simulink model "PerturbacoesOrbitais"  (R2023b)
settings: Solver=FixedStepAuto  StartTime=0.0  StopTime=tf  FixedStep=step_modelo  RelTol=1e-3
values from neighbouring files (symbols this model uses):
  J2 = 1082.63E-6    (= 0.00108263)    [constantes.m]
  mi = 3.9860044189*10^14    (= 398600441890000)    [constantes.m]
  omega_E = 7.29211585530*10^-5    (= 7.2921158553e-05)    [constantes.m]
  Re = 6378.1363*10^3    (= 6378136.3)    [constantes.m]
undefined symbols (not defined in the file or in its folder): Cd0, Cd1, drag, J2_dist, L0, L1, m0, m1
settings Model: Creator=rodri  LastModifiedBy=rodri
settings DataIOCC: SaveOutput=off  SaveTime=off
settings ModelReferenceCC: EnableRefExpFcnMdlSchedulingChecks=on

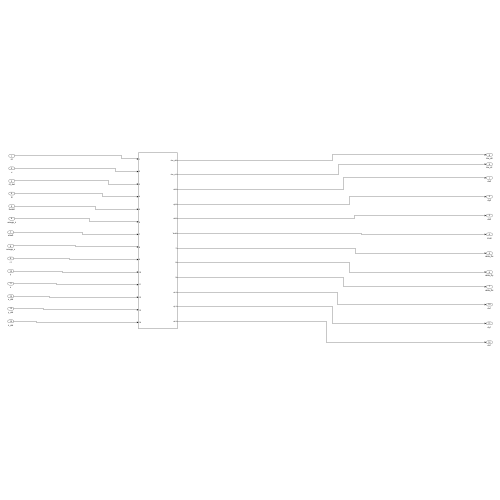
[thumbnail: Simulink's stored preview of the top-level diagram]
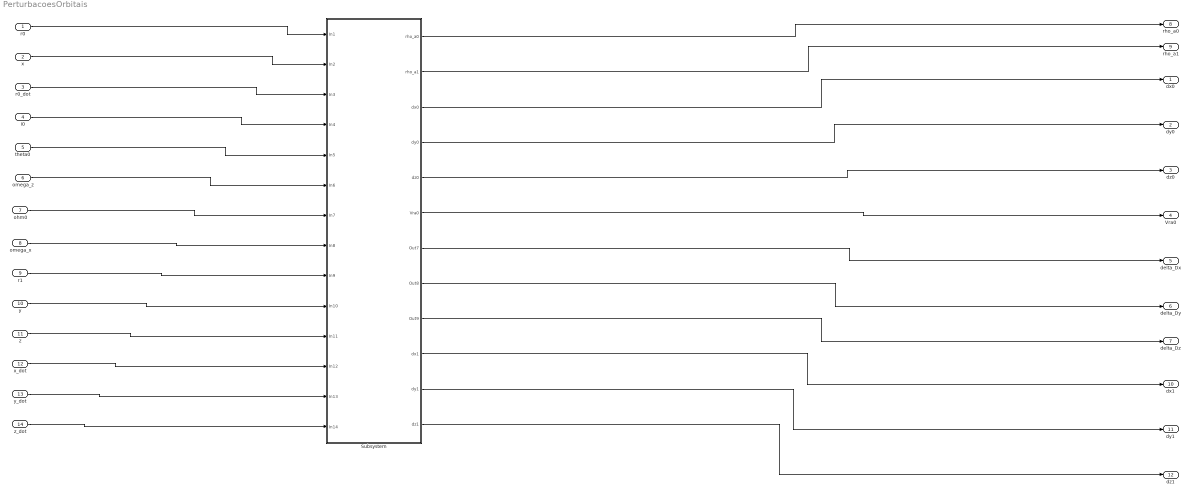
== system PerturbacoesOrbitais ==
  r0 : Inport  OutDataTypeStr=double  PortDimensions=1
  x : Inport  Port=2  OutDataTypeStr=double  PortDimensions=1
  r0_dot : Inport  Port=3  OutDataTypeStr=double  PortDimensions=1
  i0 : Inport  Port=4  OutDataTypeStr=double  PortDimensions=1
  theta0 : Inport  Port=5  OutDataTypeStr=double  PortDimensions=1
  omega_z : Inport  Port=6  OutDataTypeStr=double  PortDimensions=1
  ohm0 : Inport  Port=7  OutDataTypeStr=double  PortDimensions=1
  omega_x : Inport  Port=8  OutDataTypeStr=double  PortDimensions=1
  r1 : Inport  Port=9  OutDataTypeStr=double  PortDimensions=1
  y : Inport  Port=10  OutDataTypeStr=double  PortDimensions=1
  z : Inport  Port=11  OutDataTypeStr=double  PortDimensions=1
  x_dot : Inport  Port=12  OutDataTypeStr=double  PortDimensions=1
  y_dot : Inport  Port=13  OutDataTypeStr=double  PortDimensions=1
  z_dot : Inport  Port=14  OutDataTypeStr=double  PortDimensions=1
  Subsystem : Subsystem
  dx0 : Outport  OutDataTypeStr=double  PortDimensions=1
  dy0 : Outport  Port=2  OutDataTypeStr=double  PortDimensions=1
  dz0 : Outport  Port=3  OutDataTypeStr=double  PortDimensions=1
  Vra0 : Outport  Port=4  OutDataTypeStr=double  PortDimensions=1
  delta_Dx : Outport  Port=5  OutDataTypeStr=double  PortDimensions=1
  delta_Dy : Outport  Port=6  OutDataTypeStr=double  PortDimensions=1
  delta_Dz : Outport  Port=7  OutDataTypeStr=double  PortDimensions=1
  rho_a0 : Outport  Port=8  OutDataTypeStr=double  PortDimensions=1
  rho_a1 : Outport  Port=9  OutDataTypeStr=double  PortDimensions=1
  dx1 : Outport  Port=10  OutDataTypeStr=double  PortDimensions=1
  dy1 : Outport  Port=11  OutDataTypeStr=double  PortDimensions=1
  dz1 : Outport  Port=12  OutDataTypeStr=double  PortDimensions=1
  wires:
  r0/1 -> Subsystem/1(In1)
  x/1 -> Subsystem/2(In2)
  r0_dot/1 -> Subsystem/3(In3)
  i0/1 -> Subsystem/4(In4)
  theta0/1 -> Subsystem/5(In5)
  omega_z/1 -> Subsystem/6(In6)
  ohm0/1 -> Subsystem/7(In7)
  omega_x/1 -> Subsystem/8(In8)
  r1/1 -> Subsystem/9(In9)
  y/1 -> Subsystem/10(In10)
  z/1 -> Subsystem/11(In11)
  x_dot/1 -> Subsystem/12(In12)
  y_dot/1 -> Subsystem/13(In13)
  z_dot/1 -> Subsystem/14(In14)
  Subsystem/1(rho_a0) -> rho_a0/1
  Subsystem/2(rho_a1) -> rho_a1/1
  Subsystem/3(dx0) -> dx0/1
  Subsystem/4(dy0) -> dy0/1
  Subsystem/5(dz0) -> dz0/1
  Subsystem/6(Vra0) -> Vra0/1
  Subsystem/7(Out7) -> delta_Dx/1
  Subsystem/8(Out8) -> delta_Dy/1
  Subsystem/9(Out9) -> delta_Dz/1
  Subsystem/10(dx1) -> dx1/1
  Subsystem/11(dy1) -> dy1/1
  Subsystem/12(dz1) -> dz1/1

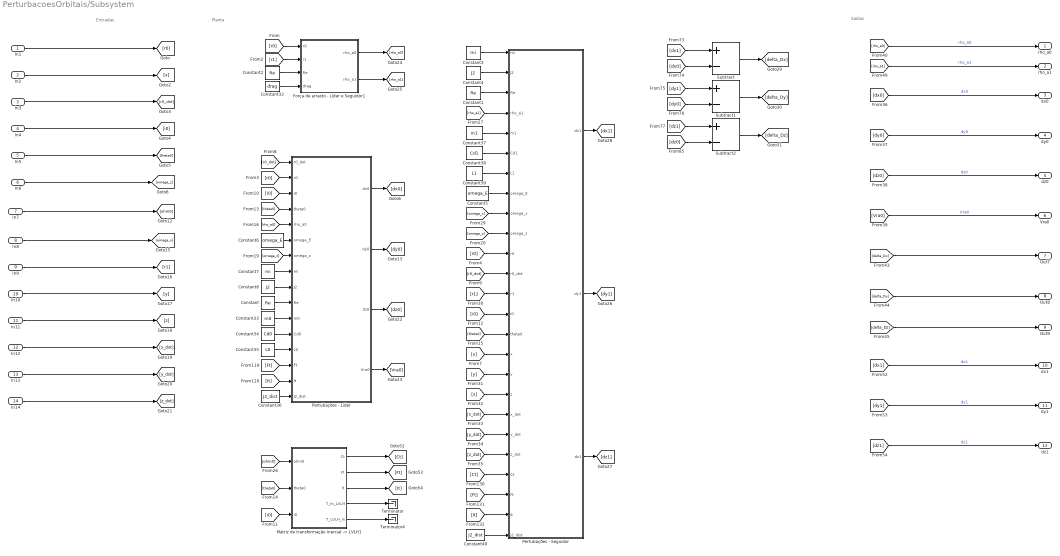
== system PerturbacoesOrbitais/Subsystem ==
  note: Planta
  note: Saídas
  note: Entradas
  In1 : Inport
  In2 : Inport  Port=2
  In3 : Inport  Port=3
  In4 : Inport  Port=4
  In5 : Inport  Port=5
  In6 : Inport  Port=6
  In7 : Inport  Port=7
  In8 : Inport  Port=8
  In9 : Inport  Port=9
  In10 : Inport  Port=10
  In11 : Inport  Port=11
  In12 : Inport  Port=12
  In13 : Inport  Port=13
  In14 : Inport  Port=14
  Constant : Constant  Value=Re
  Constant1 : Constant  Value=Re
  Constant2 : Constant  Value=Re
  Constant3 : Constant  Value=mi
  Constant32 : Constant  Value=drag  OutDataTypeStr=boolean
  Constant33 : Constant  Value=m0
  Constant34 : Constant  Value=Cd0
  Constant35 : Constant  Value=L0
  Constant36 : Constant  Value=J2_dist  OutDataTypeStr=boolean
  Constant37 : Constant  Value=m1
  Constant38 : Constant  Value=Cd1
  Constant39 : Constant  Value=L1
  Constant4 : Constant  Value=J2
  Constant40 : Constant  Value=J2_dist  OutDataTypeStr=boolean
  Constant5 : Constant  Value=omega_E
  Constant6 : Constant  Value=omega_E
  Constant7 : Constant  Value=mi
  Constant8 : Constant  Value=J2
  Força de arrasto - Líder e Seguidor1 : MATLAB Function  TreatAsAtomicUnit=on
  "Matriz de transformação Inercial -> LVLH1" : MATLAB Function  TreatAsAtomicUnit=on
  Pertubações - Líder : MATLAB Function  TreatAsAtomicUnit=on
  Pertubações - Seguidor : MATLAB Function  TreatAsAtomicUnit=on
  Subtract : Sum  Inputs=+-
  Subtract1 : Sum  Inputs=+-
  Subtract2 : Sum  Inputs=+-
  Terminator : Terminator
  Terminator4 : Terminator
  rho_a0 : Outport
  rho_a1 : Outport  Port=2
  dx0 : Outport  Port=3
  dy0 : Outport  Port=4
  dz0 : Outport  Port=5
  Vra0 : Outport  Port=6
  Out7 : Outport  Port=7
  Out8 : Outport  Port=8
  Out9 : Outport  Port=9
  dx1 : Outport  Port=10
  dy1 : Outport  Port=11
  dz1 : Outport  Port=12
  wires:
  Constant4/1 -> Pertubações - Seguidor/2(J2)
  Pertubações - Seguidor/3(dz1) -> [dz1]
  Constant6/1 -> Pertubações - Líder/6(omega_E)
  Subtract1/1 -> [delta_Dy]
  [dy0] -> dy0/1  "dy0"
  [omega_x] -> Pertubações - Seguidor/9(omega_x)
  [theta0] -> Pertubações - Seguidor/15(theta0)
  Subtract2/1 -> [delta_Dz]
  [It] -> Pertubações - Líder/15(It)
  "Matriz de transformação Inercial -> LVLH1"/5(T_LVLH_In) -> Terminator4/1
  [rho_a0] -> Pertubações - Líder/5(rho_a0)
  [y_dot] -> Pertubações - Seguidor/20(y_dot)
  [i0] -> Pertubações - Líder/3(i0)
  [z] -> Pertubações - Seguidor/18(z)
  Constant33/1 -> Pertubações - Líder/11(m0)
  Força de arrasto - Líder e Seguidor1/2(rho_a1) -> [rho_a1]
  [x] -> Pertubações - Seguidor/16(x)
  "Matriz de transformação Inercial -> LVLH1"/4(T_In_LVLH) -> Terminator/1
  "Matriz de transformação Inercial -> LVLH1"/2(Ft) -> [Ft]
  [r0] -> Pertubações - Líder/2(r0)
  Constant3/1 -> Pertubações - Seguidor/1(mi)
  [y] -> Pertubações - Seguidor/17(y)
  Constant8/1 -> Pertubações - Líder/9(J2)
  [dy1] -> Subtract1/1
  Pertubações - Seguidor/2(dy1) -> [dy1]
  In4/1 -> [i0]
  [It] -> Pertubações - Seguidor/24(It)
  [rho_a1] -> Pertubações - Seguidor/4(rho_a1)
  "Matriz de transformação Inercial -> LVLH1"/3(It) -> [It]
  [rho_a0] -> rho_a0/1  "rho_a0"
  Constant/1 -> Pertubações - Líder/10(Re)
  [r0] -> Pertubações - Seguidor/11(r0)
  Constant38/1 -> Pertubações - Seguidor/6(Cd1)
  [Ft] -> Pertubações - Líder/14(Ft)
  [dy0] -> Subtract1/2
  Constant40/1 -> Pertubações - Seguidor/25(J2_dist)
  Constant1/1 -> Pertubações - Seguidor/3(Re)
  Constant7/1 -> Pertubações - Líder/8(mi)
  [r0] -> Força de arrasto - Líder e Seguidor1/1(r0)
  "Matriz de transformação Inercial -> LVLH1"/1(Ct) -> [Ct]
  [dz1] -> Subtract2/1
  In14/1 -> [z_dot]
  [r1] -> Pertubações - Seguidor/13(r1)
  [z_dot] -> Pertubações - Seguidor/21(z_dot)
  [Ct] -> Pertubações - Seguidor/22(Ct)
  [dz0] -> Subtract2/2
  [r1] -> Força de arrasto - Líder e Seguidor1/2(r1)
  [dx0] -> Subtract/2
  Constant5/1 -> Pertubações - Seguidor/8(omega_E)
  [i0] -> "Matriz de transformação Inercial -> LVLH1"/3(i0)
  [omega_z] -> Pertubações - Seguidor/10(omega_z)
  Constant34/1 -> Pertubações - Líder/12(Cd0)
  [theta0] -> "Matriz de transformação Inercial -> LVLH1"/2(theta0)
  Pertubações - Líder/3(dz0) -> [dz0]
  Constant36/1 -> Pertubações - Líder/16(J2_dist)
  [theta0] -> Pertubações - Líder/4(theta0)
  Pertubações - Líder/2(dy0) -> [dy0]
  [x_dot] -> Pertubações - Seguidor/19(x_dot)
  [r0_dot] -> Pertubações - Seguidor/12(r0_dot)
  Subtract/1 -> [delta_Dx]
  Constant2/1 -> Força de arrasto - Líder e Seguidor1/3(Re)
  [i0] -> Pertubações - Seguidor/14(i0)
  [dx1] -> Subtract/1
  Constant39/1 -> Pertubações - Seguidor/7(L1)
  [r0_dot] -> Pertubações - Líder/1(r0_dot)
  [ohm0] -> "Matriz de transformação Inercial -> LVLH1"/1(ohm0)
  Pertubações - Líder/1(dx0) -> [dx0]
  [Ft] -> Pertubações - Seguidor/23(Ft)
  Constant32/1 -> Força de arrasto - Líder e Seguidor1/4(drag)
  Constant35/1 -> Pertubações - Líder/13(L0)
  Força de arrasto - Líder e Seguidor1/1(rho_a0) -> [rho_a0]
  Pertubações - Líder/4(Vra0) -> [Vra0]
  [dy1] -> dy1/1  "dy1"
  [delta_Dx] -> Out7/1
  Pertubações - Seguidor/1(dx1) -> [dx1]
  [omega_z] -> Pertubações - Líder/7(omega_z)
  Constant37/1 -> Pertubações - Seguidor/5(m1)
  In9/1 -> [r1]
  In12/1 -> [x_dot]
  [dz0] -> dz0/1  "dz0"
  [Vra0] -> Vra0/1  "Vra0"
  [rho_a1] -> rho_a1/1  "rho_a1"
  In3/1 -> [r0_dot]
  [dz1] -> dz1/1  "dz1"
  In11/1 -> [z]
  In1/1 -> [r0]
  [delta_Dz] -> Out9/1
  In13/1 -> [y_dot]
  In10/1 -> [y]
  [dx0] -> dx0/1  "dx0"
  In6/1 -> [omega_z]
  In2/1 -> [x]
  In5/1 -> [theta0]
  In8/1 -> [omega_x]
  [delta_Dy] -> Out8/1
  [dx1] -> dx1/1  "dx1"
  In7/1 -> [ohm0]

== matlab function PerturbacoesOrbitais/Subsystem/Matriz de transformação Inercial -> LVLH1 ==
  data: ohm0 input; Ct output; Ft output; theta0 input; i0 input; It output; T_In_LVLH output; T_LVLH_In output
function [Ct,Ft,It,T_In_LVLH,T_LVLH_In] = fcn(ohm0,theta0,i0)

[T_In_LVLH,T_LVLH_In] = TransInerLVLH(ohm0,theta0,i0);

Ct = T_In_LVLH(1,3);
Ft = T_In_LVLH(2,3);
It = T_In_LVLH(3,3);

== matlab function PerturbacoesOrbitais/Subsystem/Pertubações - Líder ==
  data: r0_dot input; dx0 output; r0 input; i0 input; theta0 input; rho_a0 input; dy0 output; dz0 output; omega_E input; omega_z input; mi input; J2 input; Re input; m0 input; Cd0 input; L0 input; Vra0 output; Ft input; It input; J2_dist input
function [dx0,dy0,dz0,Vra0] = fcn(r0_dot,r0,i0,theta0,rho_a0,omega_E,omega_z,mi,J2,Re,m0,Cd0,L0,Ft,It,J2_dist)

b0 = m0/(Cd0*(L0^2));

Vra0 = sqrt((r0_dot)^2 + (r0*omega_z - It*omega_E*r0)^2 + (Ft*omega_E*r0)^2);

if J2_dist == false
    j2 = 0;
else
    j2 = J2;
end

dx0 = ((-3*mi*j2*Re^2)/(2*r0^4))*(1 - 3*(sin(i0)^2)*(sin(theta0)^2)) - (1/2)*(rho_a0/b0)*Vra0*r0_dot*10^-2;
dy0 = ((-3*mi*j2*Re^2)/(2*r0^4))*((sin(i0)^2)*(sin(2*theta0))) - (1/2)*(rho_a0/b0)*Vra0*(r0*omega_z - It*omega_E*r0)*10^-2;
dz0 = ((-3*mi*j2*Re^2)/(2*r0^4))*(sin(theta0)*(sin(2*i0))) - (1/2)*(rho_a0/b0)*Vra0*Ft*omega_E*r0*10^-2;

== matlab function PerturbacoesOrbitais/Subsystem/Pertubações - Seguidor ==
  data: mi input; dx1 output; J2 input; Re input; rho_a1 input; m1 input; Cd1 input; L1 input; omega_E input; omega_x input; omega_z input; r0 input; r0_dot input; r1 input; i0 input; theta0 input; x input; y input; z input; x_dot input; y_dot input; z_dot input; dy1 output; dz1 output; Ct input; Ft input; It input; J2_dist input
function [dx1,dy1,dz1] = fcn(mi,J2,Re,rho_a1,m1,Cd1,L1,omega_E,omega_x,omega_z,r0,r0_dot,r1,i0,theta0,x,y,z,x_dot,y_dot,z_dot,Ct,Ft,It,J2_dist)

b1 = m1/(Cd1*((L1^2)*sqrt(2)));

if J2_dist == false
    j2 = 0;
else
    j2 = J2;
end


k2 = (r0 + x)*sin(i0)*sin(theta0) + y*cos(theta0)*sin(i0) + z*cos(i0);
k1 = (5*k2^2)/(r1^2) - 1;
k3 = (r0_dot + x_dot - omega_z*y) - (Ft*omega_E*z - y*It*omega_E);
k4 = (r0*omega_z + y_dot + omega_z*x - omega_x*z) - ((r0 + x)*It*omega_E - z*Ct*omega_E);
k5 = (z_dot + omega_x*y) - (y*Ct*omega_E - (r0 + x)*Ft*omega_E);

Vra1 = sqrt(k3^2 + k4^2 + k5^2);
dx1 = ((3*mi*j2*Re^2)/(2*(r1^5)))*(k1*(r0 + x) - 2*k2*sin(i0)*sin(theta0)) - (1/2)*(rho_a1/b1)*Vra1*k3*10^-2; %24
dy1 = ((3*mi*j2*Re^2)/(2*(r1^5)))*(k1*y - 2*k2*sin(i0)*cos(theta0)) - (1/2)*(rho_a1/b1)*Vra1*k4*10^-2; %25
dz1 = ((3*mi*j2*Re^2)/(2*(r1^5)))*(k1*z - 2*k2*cos(i0)) - (1/2)*(rho_a1/b1)*Vra1*k5*10^-2; %26

== matlab function PerturbacoesOrbitais/Subsystem/Força de arrasto - Líder e Seguidor1 ==
  data: r0 input; r1 input; rho_a0 output; rho_a1 output; Re input; drag input
function [rho_a0,rho_a1] = fcn(r0,r1,Re,drag)

if drag == false
    rho_a0 = 0;
    rho_a1 = 0;
else
    rho_a0 = densAtm(r0-Re);
    rho_a1 = densAtm(r1-Re);
end
